simulink model "Step_7"  (Simulink 7.2)
settings: Solver=ode23t  StartTime=0.0  StopTime=inf  FixedStep=0.1  MaxStep=1  RelTol=1e-3
model workspace (MAT data in the model file):
  k = 0.01
  h0 = 1
  r2h : num (value not decoded)
PreLoadFcn:
  | bdclose all
libraries: simulink x5, sfWorkshop_libs x2, gaugeslibv2 x2
settings Model: Creator=wcampbel  LastModifiedBy=wcampbel
settings OptimizationCC: InitFltsAndDblsToZero=on

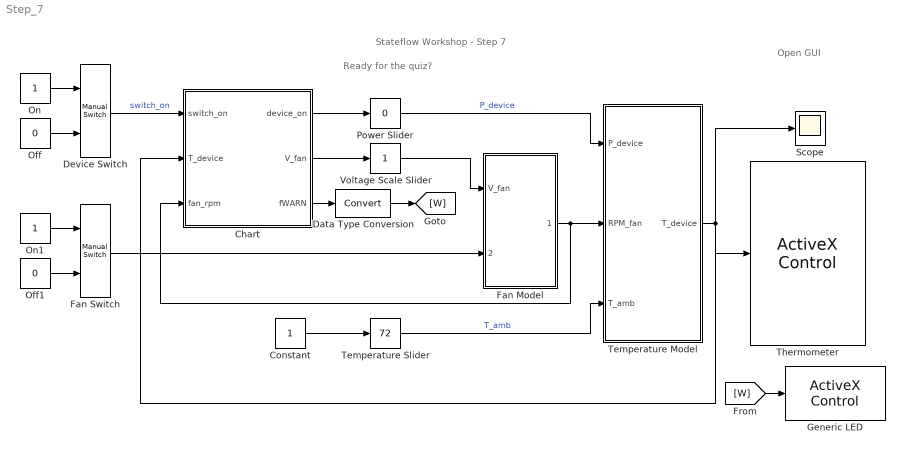
== system Step_7 ==
  note: Stateflow Workshop - Step 7
  note: Ready for the quiz?
  note: Open GUI
  Chart : Stateflow chart
  Constant : Constant  OutDataType=sfix(16)  OutScaling=2^0
  Data Type Conversion : DataTypeConversion  OutDataType=sfix(16)  OutScaling=2^0
  Device Switch : simulink/Signal Routing/Manual Switch  SystemSampleTime=-1  sw=0  action=0  varsize=off
  Fan Model : Subsystem  BlockChoice=Advanced
      settings: TemplateBlock=sfWorkshop_libs/Fan Model  MemberBlocks=Advanced,Simple
  Fan Switch : simulink/Signal Routing/Manual Switch  SystemSampleTime=-1  sw=1  action=0  varsize=off
  Generic LED : gaugeslibv2/ActiveX Control  progid=MWLED.ledctrl.1  connect=input  input=Value  inblock=on  border=on  updateParam=0
  Off : Constant  Value=0  OutDataType=sfix(16)  OutScaling=2^0
  Off1 : Constant  Value=0  OutDataType=sfix(16)  OutScaling=2^0
  On : Constant  OutDataType=sfix(16)  OutScaling=2^0
  On1 : Constant  OutDataType=sfix(16)  OutScaling=2^0
  Power Slider : simulink/Math Operations/Slider Gain  SystemSampleTime=-1  low=0  gain=0  high=400
  Scope : Scope
  Temperature Model : Subsystem  BlockChoice=(No Pace Control)
      settings: TemplateBlock=sfWorkshop_libs/Temperature Model  MemberBlocks=(No Pace Control),(Pace Control)
  Temperature Slider : simulink/Math Operations/Slider Gain  SystemSampleTime=-1  low=0  gain=72  high=110
  Thermometer : gaugeslibv2/ActiveX Control  Tag=000  progid=mwslider.sliderctrl.1  connect=input  input=Value  init=hActx.configuration='Slider\Thermometer'; hActx.MouseControl = 'NoMouseControl';  inblock=on  border=on  updateParam=0
  Voltage Scale Slider : simulink/Math Operations/Slider Gain  SystemSampleTime=-1  low=0  gain=1  high=2
  wires:
  On/1 -> Device Switch/1
  Off/1 -> Device Switch/2
  Constant/1 -> Temperature Slider/1
  Chart/2(V_fan) -> Voltage Scale Slider/1
  Temperature Model/1(T_device) -> Chart/2(T_device), Scope/1, Thermometer/1
  Power Slider/1 -> Temperature Model/1(P_device)  "P_device"
  Temperature Slider/1 -> Temperature Model/3(T_amb)  "T_amb"
  Fan Model/1(RPM_fan) -> Temperature Model/2(RPM_fan), Chart/3(fan_rpm)
  Voltage Scale Slider/1 -> Fan Model/1(V_fan)
  On1/1 -> Fan Switch/1
  Off1/1 -> Fan Switch/2
  Fan Switch/1 -> Fan Model/2(Override)
  Chart/1(device_on) -> Power Slider/1
  Device Switch/1 -> Chart/1(switch_on)  "switch_on"
  Data Type Conversion/1 -> [W]
  Chart/3(fWARN) -> Data Type Conversion/1
  [W] -> Generic LED/1

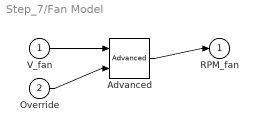
== system Step_7/Fan Model ==
  V_fan : Inport
  Override : Inport  Port=2
  Advanced : sfWorkshop_libs/Advanced  SystemSampleTime=-1
  RPM_fan : Outport
  wires:
  V_fan/1 -> Advanced/1
  Override/1 -> Advanced/2
  Advanced/1 -> RPM_fan/1

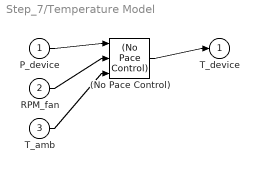
== system Step_7/Temperature Model ==
  P_device : Inport
  RPM_fan : Inport  Port=2
  T_amb : Inport  Port=3
  (No Pace Control) : sfWorkshop_libs/(No Pace Control)  SystemSampleTime=-1
  T_device : Outport
  wires:
  P_device/1 -> (No Pace Control)/1
  RPM_fan/1 -> (No Pace Control)/2
  T_amb/1 -> (No Pace Control)/3
  (No Pace Control)/1 -> T_device/1

== stateflow chart Chart ==
  state DeviceLogic [parallel]
    settings: executionOrder=1
    state DeviceOn
      entry: device_on = 1;
      during: FanTable(T_device)
    state DeviceOff
      entry: device_on = 0;
    DeviceOff -> DeviceOn : [switch_on && isCool(T_device)]
    DeviceOn -> DeviceOff : [!switch_on || !isCool(T_device)]
        | {fan_mode = 0;}
    (default) -> DeviceOff
  state status = isCool(T) [function]
    (default) -> (junction 19)
    (junction 19) -> (junction 18) [order 2] : {status = 0;}
    (junction 19) -> (junction 18) [order 1] : [T<=160]{status = 1;}
  state FanTable(T) [function]
    (default) -> (junction 20)
    (junction 20) -> (junction 21) : {
        | /* Device is cold */
        | aVarTruthTableCondition_1 = (T < 50);
        | }
    (junction 21) -> (junction 22) : {
        | /* Device is lukewarm */
        | aVarTruthTableCondition_2 = (T < 120);
        | }
    (junction 22) -> (junction 23) : {
        | /* Device is warm */
        | aVarTruthTableCondition_3 = (T < 160);
        | }
    (junction 23) -> (junction 24) [order 1] : [aVarTruthTableCondition_1]
    (junction 24) -> (junction 25) : {
        | /* 'A1':no fan (too cold or too hot) */
        | fan_mode = 0;
        | }
    (junction 23) -> (junction 26) [order 2]
    (junction 26) -> (junction 27) [order 1] : [aVarTruthTableCondition_2]
    (junction 27) -> (junction 28) : {
        | /* 'A2':low fan */
        | fan_mode = 1;
        | }
    (junction 26) -> (junction 29) [order 2]
    (junction 29) -> (junction 30) [order 1] : [aVarTruthTableCondition_3]
    (junction 30) -> (junction 31) : {
        | /* 'A3':high fan */
        | fan_mode = 2;
        | }
    (junction 29) -> (junction 32) [order 2]
    (junction 32) -> (junction 33) : /* Default */
    (junction 33) -> (junction 34) : {
        | /* 'A1':no fan (too cold or too hot) */
        | fan_mode = 0;
        | }
  state Warnings [parallel]
    settings: executionOrder=3
    state OK
    state fWARN
    (default) -> OK
    OK -> fWARN : Fevent
  state FanLogic [parallel]
    settings: executionOrder=2
    state FanSystem
      (history)
      state FanLo
        entry: V_fan[idx] = 0.75;
      state FanOff
        entry: V_fan[idx] = 0;
      state FanHi
        entry: V_fan[idx] = 1.0;
      FanLo -> FanHi [order 1] : [fan_mode == 2]
      FanHi -> FanLo [order 1] : [fan_mode == 1 && after(60,sec)]
      FanHi -> FanOff [order 2] : [fan_mode == 0]
      FanOff -> FanHi [order 2] : [fan_mode == 2]
      FanLo -> FanOff [order 2] : [fan_mode == 0 && after(60,sec)]
      FanOff -> FanLo [order 1] : [fan_mode == 1]
      (default) -> FanOff : {idx = 0;}
    FanSystem -> FanSystem : [isFanBroken(fan_mode,fan_rpm[0],t) && idx == 0]
        | {V_fan[0] = 0; idx = 1; send(Fevent,Warnings)}
  data: status function_output double; T function_input double; T function_input double; aVarTruthTableCondition_1 temporary boolean =0; aVarTruthTableCondition_2 temporary boolean =0; aVarTruthTableCondition_3 temporary boolean =0; setting function_input double; speed function_input double; busted function_output double; curTime function_input double; device_on output double; switch_on input double; T_device input double; V_fan output double size=2; fan_mode local double; fan_rpm input double; fWARN output boolean; idx local double
  data aVarTruthTableCondition_1 settings: description=Device is cold
  data aVarTruthTableCondition_2 settings: description=Device is lukewarm
  data aVarTruthTableCondition_3 settings: description=Device is warm
  events: Fevent local EITHER_EDGE_EVENT
  function busted = isFanBroken(setting,speed,curTime):
    | function busted = isFanBroken(setting,speed,curTime)
    | 
    | busted = checkFailure(setting,speed,curTime);
